simulink model "M0_PMSG_GFM_5MW_Prototype"  (R2024b)
settings: Solver=ode15s  StartTime=0  StopTime=0.2  MaxStep=2e-5  RelTol=1e-7
InitFcn:
  | m0ModelDir=fileparts(get_param(bdroot,'FileName'));if ~isempty(m0ModelDir), addpath(m0ModelDir); end
model workspace (MAT data in the model file):
  M0_pvec = [5000000; 1500; 314.159265359; 563.38264084; 0.0004761; 4.54642010436e-05; 0.000275; 0.1; 0.0019044; 7.57736684061e-05; 0.3; 1.27; 0.0005; 0.00105; 0.00105; 8.64; 20; 259.2; 11966023.932; 4960009.92002; 868001736.003; 3100006.20001; 262989.536968; 109011.207033; 7.8983182658; 8.6071416999; 1.44117647059; 1.66666557377; 0.085698; 0.897427357424; 0.0933053018116; 9.77090835708; 3; 1.25663706144e-06; 125.663706144; 9.2e-08; 5000000; 0; 4105629.37652; 556.444589246; 1; 1; 0]
  M0_x0 = [0.00472997830099; 1.27; 1.27; 0; 15839.6195082; 15839.6195082; 0; 0; 1500; 5000000; 0; 314.159265359; 0.255900963025; 0.415293030495; -0.00358787421798; 559.296822966; 0.0228860191818; 5783.5742669; 1562.8859024; 539.50087828; 136.184707222; 5795.33978098; 1516.27637252]
Description:
  | 5 MW PMSG M0 ideal continuous average model. 23 explicit continuous states; no PWM, digital delay, limiter, PLL/presynchronization, active damping, MPPT or pitch dynamics.
settings Model: Creator=Lenovo  LastModifiedBy=Lenovo
settings DataIOCC: SignalLogging=off
settings DebuggingCC: AlgebraicLoopMsg=error  UnconnectedInputMsg=error  UnconnectedOutputMsg=warning

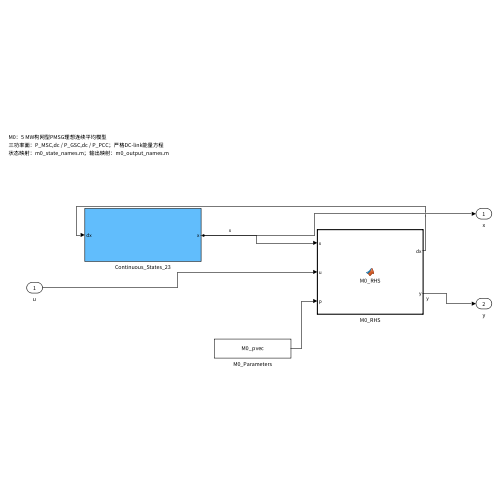
[thumbnail: Simulink's stored preview of the top-level diagram]
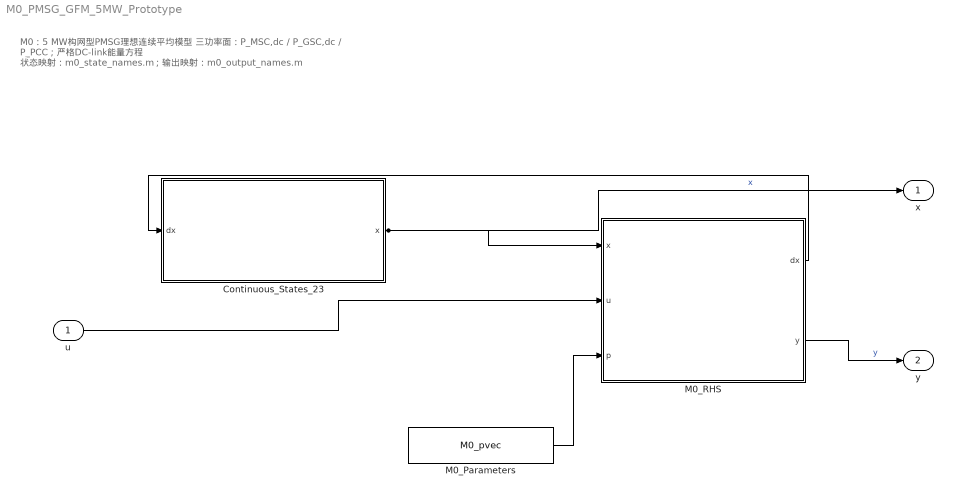
== system M0_PMSG_GFM_5MW_Prototype ==
  note: M0：5 MW构网型PMSG理想连续平均模型
      | 三功率面：P_MSC,dc / P_GSC,dc / P_PCC；严格DC-link能量方程
      | 状态映射：m0_state_names.m；输出映射：m0_output_names.m
  u : Inport  OutDataTypeStr=double  PortDimensions=6  SampleTime=0
  Continuous_States_23 : Subsystem
  M0_Parameters : Constant  Value=M0_pvec  OutDataTypeStr=double
  M0_RHS : MATLAB Function  TreatAsAtomicUnit=on
  x : Outport
  y : Outport  Port=2
  wires:
  Continuous_States_23/1(x) -> M0_RHS/1(x), x/1  "x"
  u/1 -> M0_RHS/2(u)
  M0_Parameters/1 -> M0_RHS/3(p)
  M0_RHS/1(dx) -> Continuous_States_23/1(dx)
  M0_RHS/2(y) -> y/1  "y"

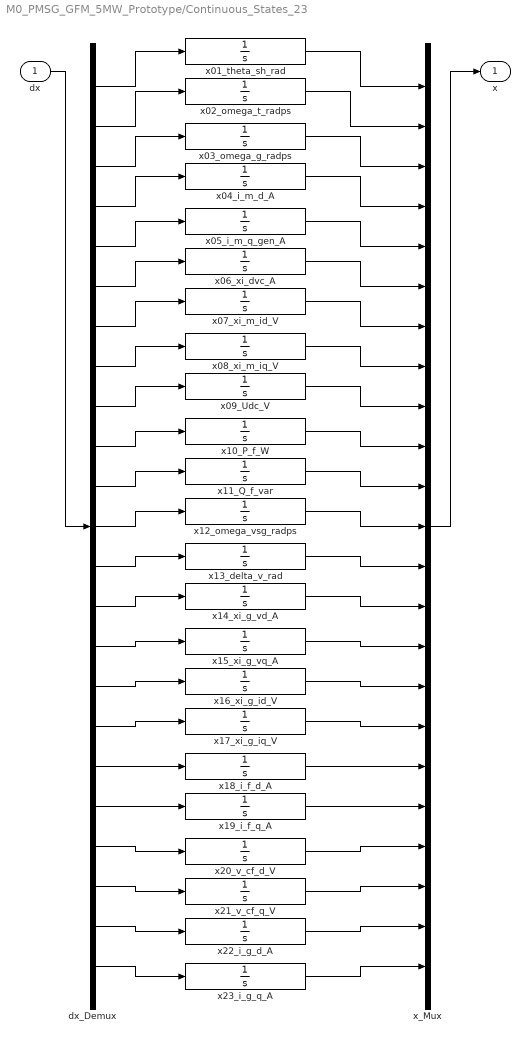
== system M0_PMSG_GFM_5MW_Prototype/Continuous_States_23 ==
  dx : Inport  PortDimensions=23
  dx_Demux : Demux  Outputs=23
  x01_theta_sh_rad : Integrator  InitialCondition=M0_x0(1)
  x02_omega_t_radps : Integrator  InitialCondition=M0_x0(2)
  x03_omega_g_radps : Integrator  InitialCondition=M0_x0(3)
  x04_i_m_d_A : Integrator  InitialCondition=M0_x0(4)
  x05_i_m_q_gen_A : Integrator  InitialCondition=M0_x0(5)
  x06_xi_dvc_A : Integrator  InitialCondition=M0_x0(6)
  x07_xi_m_id_V : Integrator  InitialCondition=M0_x0(7)
  x08_xi_m_iq_V : Integrator  InitialCondition=M0_x0(8)
  x09_Udc_V : Integrator  InitialCondition=M0_x0(9)
  x10_P_f_W : Integrator  InitialCondition=M0_x0(10)
  x11_Q_f_var : Integrator  InitialCondition=M0_x0(11)
  x12_omega_vsg_radps : Integrator  InitialCondition=M0_x0(12)
  x13_delta_v_rad : Integrator  InitialCondition=M0_x0(13)
  x14_xi_g_vd_A : Integrator  InitialCondition=M0_x0(14)
  x15_xi_g_vq_A : Integrator  InitialCondition=M0_x0(15)
  x16_xi_g_id_V : Integrator  InitialCondition=M0_x0(16)
  x17_xi_g_iq_V : Integrator  InitialCondition=M0_x0(17)
  x18_i_f_d_A : Integrator  InitialCondition=M0_x0(18)
  x19_i_f_q_A : Integrator  InitialCondition=M0_x0(19)
  x20_v_cf_d_V : Integrator  InitialCondition=M0_x0(20)
  x21_v_cf_q_V : Integrator  InitialCondition=M0_x0(21)
  x22_i_g_d_A : Integrator  InitialCondition=M0_x0(22)
  x23_i_g_q_A : Integrator  InitialCondition=M0_x0(23)
  x_Mux : Mux  Inputs=23
  x : Outport
  wires:
  dx/1 -> dx_Demux/1
  dx_Demux/1 -> x01_theta_sh_rad/1
  x01_theta_sh_rad/1 -> x_Mux/1
  dx_Demux/2 -> x02_omega_t_radps/1
  x02_omega_t_radps/1 -> x_Mux/2
  dx_Demux/3 -> x03_omega_g_radps/1
  x03_omega_g_radps/1 -> x_Mux/3
  dx_Demux/4 -> x04_i_m_d_A/1
  x04_i_m_d_A/1 -> x_Mux/4
  dx_Demux/5 -> x05_i_m_q_gen_A/1
  x05_i_m_q_gen_A/1 -> x_Mux/5
  dx_Demux/6 -> x06_xi_dvc_A/1
  x06_xi_dvc_A/1 -> x_Mux/6
  dx_Demux/7 -> x07_xi_m_id_V/1
  x07_xi_m_id_V/1 -> x_Mux/7
  dx_Demux/8 -> x08_xi_m_iq_V/1
  x08_xi_m_iq_V/1 -> x_Mux/8
  dx_Demux/9 -> x09_Udc_V/1
  x09_Udc_V/1 -> x_Mux/9
  dx_Demux/10 -> x10_P_f_W/1
  x10_P_f_W/1 -> x_Mux/10
  dx_Demux/11 -> x11_Q_f_var/1
  x11_Q_f_var/1 -> x_Mux/11
  dx_Demux/12 -> x12_omega_vsg_radps/1
  x12_omega_vsg_radps/1 -> x_Mux/12
  dx_Demux/13 -> x13_delta_v_rad/1
  x13_delta_v_rad/1 -> x_Mux/13
  dx_Demux/14 -> x14_xi_g_vd_A/1
  x14_xi_g_vd_A/1 -> x_Mux/14
  dx_Demux/15 -> x15_xi_g_vq_A/1
  x15_xi_g_vq_A/1 -> x_Mux/15
  dx_Demux/16 -> x16_xi_g_id_V/1
  x16_xi_g_id_V/1 -> x_Mux/16
  dx_Demux/17 -> x17_xi_g_iq_V/1
  x17_xi_g_iq_V/1 -> x_Mux/17
  dx_Demux/18 -> x18_i_f_d_A/1
  x18_i_f_d_A/1 -> x_Mux/18
  dx_Demux/19 -> x19_i_f_q_A/1
  x19_i_f_q_A/1 -> x_Mux/19
  dx_Demux/20 -> x20_v_cf_d_V/1
  x20_v_cf_d_V/1 -> x_Mux/20
  dx_Demux/21 -> x21_v_cf_q_V/1
  x21_v_cf_q_V/1 -> x_Mux/21
  dx_Demux/22 -> x22_i_g_d_A/1
  x22_i_g_d_A/1 -> x_Mux/22
  dx_Demux/23 -> x23_i_g_q_A/1
  x23_i_g_q_A/1 -> x_Mux/23
  x_Mux/1 -> x/1

== matlab function M0_PMSG_GFM_5MW_Prototype/M0_RHS ==
  data: x input; dx output; u input; y output; p input
function [dx,y] = M0_RHS(x,u,p)
%#codegen
dx = zeros(23,1);
y = zeros(29,1);
[dx,y] = m0_nonlinear_dynamics(x,u,p);
end
